simulink model "ordre2ana"  (R2014a)
settings: Solver=ode1  StartTime=0.0  StopTime=0.004  FixedStep=Delta  RelTol=1e-3
undefined symbols (not defined in the file): F0, m, Omega
settings Model: Creator=aymeric  LastModifiedBy=aymeric

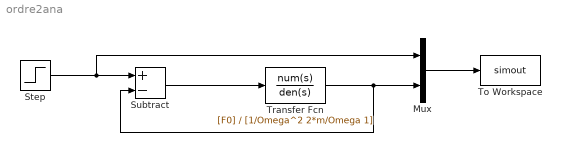
== system ordre2ana ==
  Mux : Mux  Inputs=2
  Step : Step  Time=0  SampleTime=0
  Subtract : Sum  Inputs=+-
  To Workspace : ToWorkspace  VariableName=simout  SaveFormat=Timeseries  SampleTime=-1
  Transfer Fcn : TransferFcn  Numerator=[F0]  Denominator=[1/Omega^2 2*m/Omega 1]
  wires:
  Subtract/1 -> Transfer Fcn/1
  Transfer Fcn/1 -> Mux/2, Subtract/2
  Step/1 -> Mux/1, Subtract/1
  Mux/1 -> To Workspace/1
